simulink library "findPositions_cl"  (R2018b)
settings: Solver=VariableStepAuto  StartTime=0.0  StopTime=10.0  RelTol=1e-3
libraries: findDotPositions_ul x1, findPosition_ul x1
settings Model: Creator=MAE-NCSUCORE  LastModifiedBy=MAE-NCSUCORE

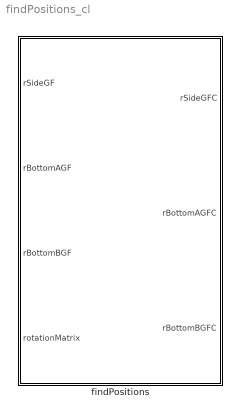
== system findPositions_cl ==
  findPositions : Subsystem  mask{rSideBF=[0; 0; 0], rBottomABF=[0; 0; 0], rBottomBBF=[0; 0; 0]}
      mask prompts: rSideBF "Vector from Side Dot Centroid to COM [cm]"; rBottomABF "Vector from Bottom A Dot Centroid to COM [cm]"; rBottomBBF "Vector from Bottom B Dot Centroid to COM [cm]"

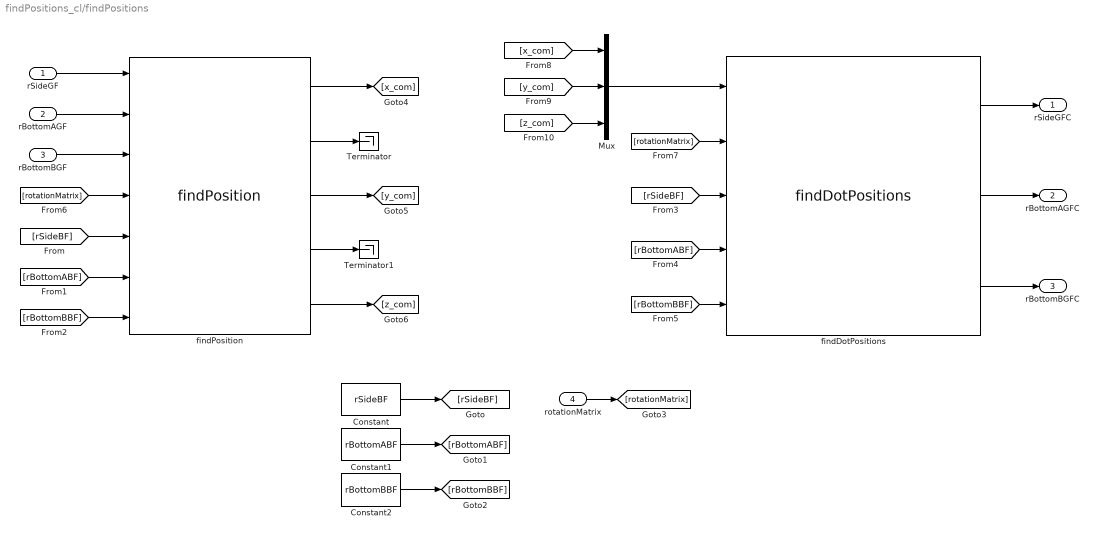
== system findPositions_cl/findPositions ==
  rSideGF : Inport
  rBottomAGF : Inport  Port=2
  rBottomBGF : Inport  Port=3
  rotationMatrix : Inport  Port=4
  Constant : Constant  Value=rSideBF
  Constant1 : Constant  Value=rBottomABF
  Constant2 : Constant  Value=rBottomBBF
  Mux : Mux  Inputs=3
  Terminator : Terminator
  Terminator1 : Terminator
  findDotPositions : findDotPositions_ul/findDotPositions  SystemSampleTime=-1
  findPosition : findPosition_ul/findPosition  SystemSampleTime=-1
  rSideGFC : Outport
  rBottomAGFC : Outport  Port=2
  rBottomBGFC : Outport  Port=3
  wires:
  [rotationMatrix] -> findDotPositions/2
  [rBottomABF] -> findDotPositions/4
  findDotPositions/1 -> rSideGFC/1
  [rBottomBBF] -> findDotPositions/5
  [rSideBF] -> findDotPositions/3
  findDotPositions/3 -> rBottomBGFC/1
  findDotPositions/2 -> rBottomAGFC/1
  Constant/1 -> [rSideBF]
  Constant1/1 -> [rBottomABF]
  Constant2/1 -> [rBottomBBF]
  [rSideBF] -> findPosition/5
  [rBottomBBF] -> findPosition/7
  [rBottomABF] -> findPosition/6
  rotationMatrix/1 -> [rotationMatrix]
  [rotationMatrix] -> findPosition/4
  findPosition/1 -> [x_com]
  findPosition/3 -> [y_com]
  findPosition/5 -> [z_com]
  [z_com] -> Mux/3
  [y_com] -> Mux/2
  [x_com] -> Mux/1
  Mux/1 -> findDotPositions/1
  findPosition/2 -> Terminator/1
  findPosition/4 -> Terminator1/1
  rSideGF/1 -> findPosition/1
  rBottomAGF/1 -> findPosition/2
  rBottomBGF/1 -> findPosition/3
